simulink model "momentumBasedFlying"  (R2021b)
settings: Solver=FixedStepAuto  StartTime=0.0  StopTime=Config.simulationTime  FixedStep=Config.tStep  RelTol=1e-3
InitFcn:
  | cd(fileparts(which(bdroot)));
  | initMomentumBasedFlying;
StopFcn:
  | cd(fileparts(which(bdroot)));
  | stopMomentumBasedFlying;
undefined symbols (not defined in the file or in its folder): biasVectorConstraint_feet, Config, confVisualizer, ConstraintMatrix_feet, DiscIntNeverNeededParam, jets_config
libraries: WBToolboxLibrary x75
(part 2 of 4)

== system momentumBasedFlying/FLYING CONTROLLER (CORE) V2.5/Flight Controller RAL-HUMANOIDS V3.1- Aerodynamic Effects Compensation/Momentum Control for Flying ==
  stateMachineQuantitites : Inport
  gainsAndReferences : Inport  Port=2
  systemState : Inport  Port=3
  kinematics : Inport  Port=4
  dynamics : Inport  Port=5
  aerodynamic_force : Inport  Port=6
  Bus Selector : BusSelector  OutputSignals=jetsIntensities
  Feedback linearization : Subsystem
  Momentum Control : Subsystem
  QP Solver and Integrate Contact Forces Derivative : Subsystem
  extendedKalmanFilter4jets : Subsystem
  jointVel_star : Outport  VectorParamsAs1DForOutWhenUnconnected=off
  contactForces_star : Outport  Port=2  VectorParamsAs1DForOutWhenUnconnected=off
  jetsIntensitiesDot_star : Outport  Port=3  VectorParamsAs1DForOutWhenUnconnected=off
  "jets_throttle " : Outport  Port=4  VectorParamsAs1DForOutWhenUnconnected=off
  wires:
  QP Solver and Integrate Contact Forces Derivative/3(jointVel_star) -> jointVel_star/1
  QP Solver and Integrate Contact Forces Derivative/1(contactForces_star) -> contactForces_star/1, Momentum Control/1(contactForces_hat)  "WARNING! estimated contact forces are assumed to be coincident with contactForces_star"
  Momentum Control/4(uppeBoundQP) -> QP Solver and Integrate Contact Forces Derivative/4(upperBoundQP)
  Momentum Control/3(lowerBoundQP) -> QP Solver and Integrate Contact Forces Derivative/3(lowerBoundQP)
  Momentum Control/2(gVectorQP) -> QP Solver and Integrate Contact Forces Derivative/2(gVectorQP)
  Momentum Control/1(HessianMatrixQP) -> QP Solver and Integrate Contact Forces Derivative/1(HessianMatrixQP)
  stateMachineQuantitites/1 -> QP Solver and Integrate Contact Forces Derivative/5(stateMachineQuantities), Momentum Control/6(stateMachineQuantitites)
  gainsAndReferences/1 -> Momentum Control/5(gainsAndReferences)
  dynamics/1 -> Momentum Control/4(dynamics)
  kinematics/1 -> Momentum Control/3(kinematics)
  systemState/1 -> Bus Selector/1, QP Solver and Integrate Contact Forces Derivative/6(systemState), Momentum Control/2(systemState)
  Feedback linearization/1(throttle) -> extendedKalmanFilter4jets/2("jetsThrottle "), "jets_throttle "/1
  Bus Selector/1 -> extendedKalmanFilter4jets/1("jetsIntensityMeasured ")  "<jetsIntensities>"
  extendedKalmanFilter4jets/1(jetsState) -> Feedback linearization/1(jetState)
  QP Solver and Integrate Contact Forces Derivative/2(jetsIntensitiesDot_star) -> jetsIntensitiesDot_star/1, Feedback linearization/2(jetDerivatives_des)
  aerodynamic_force/1 -> Momentum Control/7(aerodynamic_force)

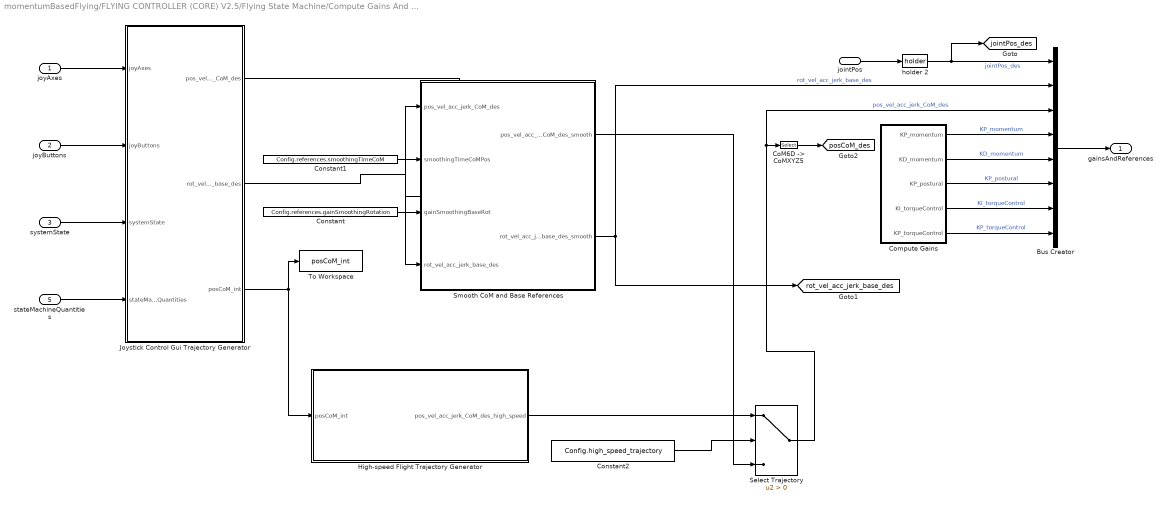
== system momentumBasedFlying/FLYING CONTROLLER (CORE) V2.5/Flying State Machine/Compute Gains And References ==
  joyAxes : Inport
  joyButtons : Inport  Port=2
  systemState : Inport  Port=3
  jointPos : Inport  Port=4
  stateMachineQuantities : Inport  Port=5
  Bus Creator : BusCreator  Inputs=8
  "CoM6D -> CoMXYZ5" : Selector  NumberOfDimensions=2  InputPortWidth=7  IndexOptions=Index vector (dialog),Index vector (dialog)  Indices=[1 2 3],[1]  OutputSizes=1,1
  Compute Gains : Subsystem
  Constant : Constant  Value=Config.references.gainSmoothingRotation
  Constant1 : Constant  Value=Config.references.smoothingTimeCoM
  Constant2 : Constant  Value=Config.high_speed_trajectory
  High-speed Flight Trajectory Generator : Subsystem
  Joystick Control Gui Trajectory Generator : Subsystem
  Select Trajectory : Switch  Criteria=u2 > Threshold
  Smooth CoM and Base References : Subsystem
  To Workspace : ToWorkspace  VariableName=posCoM_int  SaveFormat=Timeseries  SampleTime=-1
  holder 2 : WBToolboxLibrary/Utilities/holder 
      settings: SourceProductName=WholeBodyToolbox
  gainsAndReferences : Outport  VectorParamsAs1DForOutWhenUnconnected=off
  tag scope: jointPos_des=global, posCoM_des=global, rot_vel_acc_jerk_base_des=global
  wires:
  "CoM6D -> CoMXYZ5"/1 -> [posCoM_des]
  Constant1/1 -> Smooth CoM and Base References/2(smoothingTimeCoMPos)
  Smooth CoM and Base References/2(rot_vel_acc_jerk_base_des_smooth) -> [rot_vel_acc_jerk_base_des], Bus Creator/2  "rot_vel_acc_jerk_base_des"
  Compute Gains/5(KP_torqueControl) -> Bus Creator/8  "KP_torqueControl"
  Compute Gains/2(KD_momentum) -> Bus Creator/5  "KD_momentum"
  Compute Gains/1(KP_momentum) -> Bus Creator/4  "KP_momentum"
  Compute Gains/3(KP_postural) -> Bus Creator/6  "KP_postural"
  Constant/1 -> Smooth CoM and Base References/3(gainSmoothingBaseRot)
  Bus Creator/1 -> gainsAndReferences/1
  Compute Gains/4(KI_torqueControl) -> Bus Creator/7  "KI_torqueControl"
  holder 2/1 -> Bus Creator/1, [jointPos_des]  "jointPos_des"
  jointPos/1 -> holder 2/1
  joyAxes/1 -> Joystick Control Gui Trajectory Generator/1(joyAxes)
  joyButtons/1 -> Joystick Control Gui Trajectory Generator/2(joyButtons)
  systemState/1 -> Joystick Control Gui Trajectory Generator/3(systemState)
  stateMachineQuantities/1 -> Joystick Control Gui Trajectory Generator/4(stateMachineQuantities)
  Joystick Control Gui Trajectory Generator/1(pos_vel_acc_jerk_CoM_des) -> Smooth CoM and Base References/1(pos_vel_acc_jerk_CoM_des)
  Joystick Control Gui Trajectory Generator/2(rot_vel_acc_jerk_base_des) -> Smooth CoM and Base References/4(rot_vel_acc_jerk_base_des)
  High-speed Flight Trajectory Generator/1(pos_vel_acc_jerk_CoM_des_high_speed) -> Select Trajectory/1
  Smooth CoM and Base References/1(pos_vel_acc_jerk_CoM_des_smooth) -> Select Trajectory/3
  Constant2/1 -> Select Trajectory/2
  Select Trajectory/1 -> Bus Creator/3, "CoM6D -> CoMXYZ5"/1  "pos_vel_acc_jerk_CoM_des"
  Joystick Control Gui Trajectory Generator/3(posCoM_int) -> To Workspace/1, High-speed Flight Trajectory Generator/1(posCoM_int)

== system momentumBasedFlying/FLYING CONTROLLER (CORE) V2.5/Flying State Machine/Take Off//Landing State Detector ==
  systemState : Inport
  joyButtons : Inport  Port=2
  Bus Creator : BusCreator  Inputs=6
  Bus Selector : BusSelector  OutputSignals=contactForces
  Demux : Demux  Outputs=[6;6]
  MATLAB Function : MATLAB Function  TreatAsAtomicUnit=on
  Vertical Forces Control : MATLAB Function  TreatAsAtomicUnit=on
  stateMachineQuantities : Outport  VectorParamsAs1DForOutWhenUnconnected=off
  tag scope: stateMachineQuantities=global
  wires:
  Vertical Forces Control/1(decreaseMaxFootVerticalForce) -> Bus Creator/1  "decreaseMaxFootVerticalForce"
  Vertical Forces Control/2(increaseMinFootVerticalForce) -> Bus Creator/2  "increaseMinFootVerticalForce"
  Bus Creator/1 -> [stateMachineQuantities], stateMachineQuantities/1
  systemState/1 -> Bus Selector/1
  joyButtons/1 -> Vertical Forces Control/1(joyButtons)
  Demux/2 -> MATLAB Function/2(wrench_r)
  Demux/1 -> MATLAB Function/1(wrench_l)
  Bus Selector/1 -> Demux/1  "<contactForces>"
  MATLAB Function/1(feetContactIsActive) -> Bus Creator/4  "feetContactIsActive"
  MATLAB Function/2(robotIsLanded) -> Bus Creator/5  "robotIsLanded"
  MATLAB Function/3(oneFootIsInContact) -> Bus Creator/6  "oneFootIsInContact"
  Vertical Forces Control/3(activateEqConstrTorqueControl) -> Bus Creator/3  "activateEqConstrTorqueControl"

== system momentumBasedFlying/FLYING CONTROLLER (CORE) V2.5/Get System State/Change Contact Forces Representation ==
  jointPos : Inport
  w_H_b : Inport  Port=2
  contactForces_WBD : Inport  Port=3
  Change Contact Forces Representation : MATLAB Function  TreatAsAtomicUnit=on
  "CoM6D -> CoMXYZ1" : Selector  NumberOfDimensions=2  InputPortWidth=7  IndexOptions=Index vector (dialog),Index vector (dialog)  Indices=[1 2 3],[1 2 3]  OutputSizes=1,1
  "CoM6D -> CoMXYZ3" : Selector  NumberOfDimensions=2  InputPortWidth=7  IndexOptions=Index vector (dialog),Index vector (dialog)  Indices=[1 2 3],[1 2 3]  OutputSizes=1,1
  LFoot Pose : WBToolboxLibrary/Model/Kinematics/ForwardKinematics  frameName=Frames.LFOOT_FRAME
      settings: SourceProductName=WholeBodyToolbox
  Mux : Mux  Inputs=2
  RFoot Pose : WBToolboxLibrary/Model/Kinematics/ForwardKinematics  frameName=Frames.RFOOT_FRAME
      settings: SourceProductName=WholeBodyToolbox
  contactForces : Outport  VectorParamsAs1DForOutWhenUnconnected=off
  tag scope: wrench_LFoot=global, wrench_RFoot=global
  wires:
  contactForces_WBD/1 -> Change Contact Forces Representation/1(contactForces_WBD)
  RFoot Pose/1 -> "CoM6D -> CoMXYZ3"/1
  "CoM6D -> CoMXYZ3"/1 -> Change Contact Forces Representation/3(w_R_r_sole)
  LFoot Pose/1 -> "CoM6D -> CoMXYZ1"/1
  "CoM6D -> CoMXYZ1"/1 -> Change Contact Forces Representation/2(w_R_l_sole)
  w_H_b/1 -> LFoot Pose/1, RFoot Pose/1
  jointPos/1 -> LFoot Pose/2, RFoot Pose/2
  Change Contact Forces Representation/1(mixed_f_l_sole) -> [wrench_LFoot], Mux/1
  Change Contact Forces Representation/2(mixed_f_r_sole) -> [wrench_RFoot], Mux/2
  Mux/1 -> contactForces/1

== system momentumBasedFlying/Visualizer/Task and Base Frame Kinematics/Combine Rotations ==
  roll : Inport
  pitch : Inport  Port=2
  yaw : Inport  Port=3
  roll_des : Inport  Port=4
  pitch_des : Inport  Port=5
  yaw_des : Inport  Port=6
  Mux : Mux  Inputs=2
  Mux1 : Mux  Inputs=2
  Mux2 : Mux  Inputs=2
  Task rotation combined : Scope  NumInputPorts=3
  wires:
  yaw_des/1 -> Mux2/2
  pitch_des/1 -> Mux1/2
  pitch/1 -> Mux1/1
  roll/1 -> Mux/1
  yaw/1 -> Mux2/1
  roll_des/1 -> Mux/2
  Mux2/1 -> Task rotation combined/3
  Mux1/1 -> Task rotation combined/2
  Mux/1 -> Task rotation combined/1

== system momentumBasedFlying/iRonCub/Forward Dynamics/aerodynamic visualizer ==
  aerodynamic_forces_total : Inport
  relative_velocity : Inport  Port=2
  alpha : Inport  Port=3
  beta : Inport  Port=4
  drag_force : Inport  Port=5
  normal_force : Inport  Port=6
  Scope : Scope
  Scope1 : Scope
  Scope2 : Scope
  To Workspace : ToWorkspace  VariableName=Fa_drag  SaveFormat=Timeseries  SampleTime=-1
  To Workspace1 : ToWorkspace  VariableName=Fa_normal  SaveFormat=Timeseries  SampleTime=-1
  To Workspace2 : ToWorkspace  VariableName=Fa  SaveFormat=Timeseries  SampleTime=-1
  To Workspace3 : ToWorkspace  VariableName=Va  SaveFormat=Timeseries  SampleTime=-1
  To Workspace4 : ToWorkspace  VariableName=alpha  SaveFormat=Timeseries  SampleTime=-1
  To Workspace5 : ToWorkspace  VariableName=beta  SaveFormat=Timeseries  SampleTime=-1
  r : Scope
  wires:
  beta/1 -> Scope2/1, To Workspace5/1
  relative_velocity/1 -> r/1, To Workspace3/1
  aerodynamic_forces_total/1 -> Scope1/1, To Workspace2/1
  alpha/1 -> Scope/1, To Workspace4/1
  drag_force/1 -> To Workspace/1
  normal_force/1 -> To Workspace1/1

== system momentumBasedFlying/FLYING CONTROLLER (CORE) V2.5/Dynamics and Kinematics/Dynamic Quantities/Compute Centroidal Inertia ==
  M : Inport
  w_H_b : Inport  Port=2
  posCoM : Inport  Port=3
  Compute Centroidal Inertia : MATLAB Function  TreatAsAtomicUnit=on
  Selector : Selector  NumberOfDimensions=2  InputPortWidth=3  IndexOptions=Index vector (dialog),Index vector (dialog)  Indices=[1 2 3],4  OutputSizes=1,1
  w_I_c : Outport  VectorParamsAs1DForOutWhenUnconnected=off
  wires:
  M/1 -> Compute Centroidal Inertia/1(M)
  w_H_b/1 -> Selector/1
  Selector/1 -> Compute Centroidal Inertia/3(posBase)
  posCoM/1 -> Compute Centroidal Inertia/2(posCoM)
  Compute Centroidal Inertia/1(w_I_c) -> w_I_c/1

== system momentumBasedFlying/FLYING CONTROLLER (CORE) V2.5/Dynamics and Kinematics/Dynamic Quantities/Momentum and CentroidalMomentum Matrix ==
  w_H_b : Inport
  jointPos : Inport  Port=2
  w_baseTwist : Inport  Port=3
  jointVel : Inport  Port=4
  CentroidalMomentum : WBToolboxLibrary/Model/Dynamics/CentroidalMomentum
      settings: SourceProductName=WholeBodyToolbox
  CentroidalMomentum Matrix iCub 23/25 DoFs : Subsystem
  L : Outport  VectorParamsAs1DForOutWhenUnconnected=off
  CMM : Outport  Port=2  VectorParamsAs1DForOutWhenUnconnected=off
  wires:
  w_baseTwist/1 -> CentroidalMomentum/3
  CentroidalMomentum/1 -> L/1
  w_H_b/1 -> CentroidalMomentum Matrix iCub 23/25 DoFs/1(w_H_b), CentroidalMomentum/1
  jointPos/1 -> CentroidalMomentum Matrix iCub 23/25 DoFs/2(jointPos), CentroidalMomentum/2
  jointVel/1 -> CentroidalMomentum/4
  CentroidalMomentum Matrix iCub 23/25 DoFs/1(CMM) -> CMM/1

== system momentumBasedFlying/FLYING CONTROLLER (CORE) V2.5/Dynamics and Kinematics/Kinematic Quantities/Compute Thrusts Axes and Arms ==
  posCoM : Inport
  w_H_b : Inport  Port=2
  jointPos : Inport  Port=3
  Pose Jet 1 : WBToolboxLibrary/Model/Kinematics/ForwardKinematics  frameName=Frames.JET1_FRAME
      settings: SourceProductName=WholeBodyToolbox
  Pose Jet 2 : WBToolboxLibrary/Model/Kinematics/ForwardKinematics  frameName=Frames.JET2_FRAME
      settings: SourceProductName=WholeBodyToolbox
  Pose Jet 3 : WBToolboxLibrary/Model/Kinematics/ForwardKinematics  frameName=Frames.JET3_FRAME
      settings: SourceProductName=WholeBodyToolbox
  Pose Jet 4 : WBToolboxLibrary/Model/Kinematics/ForwardKinematics  frameName=Frames.JET4_FRAME
      settings: SourceProductName=WholeBodyToolbox
  Thrust Axes and Arms : MATLAB Function  TreatAsAtomicUnit=on
  matrixOfJetsAxes : Outport  VectorParamsAs1DForOutWhenUnconnected=off
  matrixOfJetsArms : Outport  Port=2  VectorParamsAs1DForOutWhenUnconnected=off
  wires:
  Pose Jet 2/1 -> Thrust Axes and Arms/2(w_H_J2)
  jointPos/1 -> Pose Jet 1/2, Pose Jet 2/2, Pose Jet 3/2, Pose Jet 4/2
  Pose Jet 1/1 -> Thrust Axes and Arms/1(w_H_J1)
  Pose Jet 3/1 -> Thrust Axes and Arms/3(w_H_J3)
  Pose Jet 4/1 -> Thrust Axes and Arms/4(w_H_J4)
  Thrust Axes and Arms/1(matrixOfJetsAxes) -> matrixOfJetsAxes/1
  Thrust Axes and Arms/2(matrixOfJetsArms) -> matrixOfJetsArms/1
  w_H_b/1 -> Pose Jet 4/1, Pose Jet 3/1, Pose Jet 2/1, Pose Jet 1/1
  posCoM/1 -> Thrust Axes and Arms/5(posCoM)

== system momentumBasedFlying/FLYING CONTROLLER (CORE) V2.5/Flight Controller RAL-HUMANOIDS V3.1- Aerodynamic Effects Compensation/Joint Torque Control for Flying/Integrate Joints Velocity error ==
  jointVel_err : Inport
  Constant : Constant  Value=zeros(Config.N_DOF,1)
  Discrete-Time Integrator1 : DiscreteIntegrator  InitialConditionSource=external  InitialCondition=zeros(Config.N_DOF,1)  SampleTime=Config.tStep  ICPrevOutput=DiscIntNeverNeededParam  ICPrevScaledInput=DiscIntNeverNeededParam
  jointPos_err : Outport  VectorParamsAs1DForOutWhenUnconnected=off
  tag scope: jointPos_err_integral=global
  wires:
  Constant/1 -> Discrete-Time Integrator1/2
  jointVel_err/1 -> Discrete-Time Integrator1/1
  Discrete-Time Integrator1/1 -> [jointPos_err_integral], jointPos_err/1

== system momentumBasedFlying/FLYING CONTROLLER (CORE) V2.5/Flight Controller RAL-HUMANOIDS V3.1- Aerodynamic Effects Compensation/Joint Torque Control for Flying/QP torqueControl ==
  HessianMatrixQP : Inport
  gVectorQP : Inport  Port=2
  ConstraintMatrix_inequality : Inport  Port=3
  biasVectorConstraint_inequality : Inport  Port=4
  feetContactIsActive : Inport  Port=5
  Constant2 : Constant  Value=Config.sat.jointTorquesSaturation
  NOT : Logic  Operator=NOT  IconShape=distinctive  AllPortsSameDT=off  OutDataTypeStr=boolean
  Process QP Inputs Torque Control : MATLAB Function  TreatAsAtomicUnit=on
  QP torqueControl - balancing : Subsystem  TreatAsAtomicUnit=on
  QP torqueControl - flight : Subsystem  TreatAsAtomicUnit=on
  Select QP torqueControl Output : Subsystem
  jointTorques_star : Outport  VectorParamsAs1DForOutWhenUnconnected=off
  exitFlagQP_torqueControl : Outport  Port=2  VectorParamsAs1DForOutWhenUnconnected=off
  wires:
  Select QP torqueControl Output/1(jointTorques_star) -> jointTorques_star/1
  Select QP torqueControl Output/2(exitFlagQP_torqueControl) -> exitFlagQP_torqueControl/1
  QP torqueControl - flight/1(QPStatus_flight) -> Select QP torqueControl Output/4(QPStatus_flight)
  QP torqueControl - flight/2(QPOutput_flight) -> Select QP torqueControl Output/5(QPOutput_flight)
  QP torqueControl - balancing/2(QPOutput_balancing) -> Select QP torqueControl Output/2(QPOutput_balancing)
  QP torqueControl - balancing/1(QPStatus_balancing) -> Select QP torqueControl Output/1(QPStatus_balancing)
  Process QP Inputs Torque Control/1(H_balancing) -> QP torqueControl - balancing/1(H)
  Process QP Inputs Torque Control/2(g_balancing) -> QP torqueControl - balancing/2(g)
  Process QP Inputs Torque Control/3(ub_balancing) -> QP torqueControl - balancing/3(ub)
  Process QP Inputs Torque Control/4(lb_balancing) -> QP torqueControl - balancing/4(lb)
  Process QP Inputs Torque Control/5(Aeq_balancing) -> QP torqueControl - balancing/5(AEq)
  Process QP Inputs Torque Control/6(lbEq_balancing) -> QP torqueControl - balancing/6(lbEq)
  Process QP Inputs Torque Control/7(ubEq_balancing) -> QP torqueControl - balancing/7(ubEq)
  Process QP Inputs Torque Control/11(lb_flight) -> QP torqueControl - flight/4(lb)
  Process QP Inputs Torque Control/10(ub_flight) -> QP torqueControl - flight/3(ub)
  Process QP Inputs Torque Control/9(g_flight) -> QP torqueControl - flight/2(g)
  Process QP Inputs Torque Control/8(H_flight) -> QP torqueControl - flight/1(H)
  Constant2/1 -> Process QP Inputs Torque Control/5(jointTorquesSaturation)
  gVectorQP/1 -> Process QP Inputs Torque Control/2(gVectorQP)
  HessianMatrixQP/1 -> Process QP Inputs Torque Control/1(HessianMatrixQP)
  ConstraintMatrix_inequality/1 -> Process QP Inputs Torque Control/3(InequalityConstrMatrix)
  biasVectorConstraint_inequality/1 -> Process QP Inputs Torque Control/4(biasVectorInequalityConstr)
  NOT/1 -> QP torqueControl - flight/Enable
  feetContactIsActive/1 -> NOT/1, QP torqueControl - balancing/Enable, Select QP torqueControl Output/3(feetContactIsActive)

== system momentumBasedFlying/FLYING CONTROLLER (CORE) V2.5/Flight Controller RAL-HUMANOIDS V3.1- Aerodynamic Effects Compensation/Joint Torque Control for Flying/Torque Derivative Saturation ==
  jointTorques_star : Inport
  Constant1 : Constant  Value=Config.tStep
  Constant2 : Constant  Value=Config.sat.jointTorquesDotMax
  Saturate Torque Derivative : MATLAB Function  TreatAsAtomicUnit=on
  "holder " : WBToolboxLibrary/Utilities/holder 
      settings: SourceProductName=WholeBodyToolbox
  jointTorques_star_sat : Outport  VectorParamsAs1DForOutWhenUnconnected=off
  wires:
  Constant2/1 -> Saturate Torque Derivative/4(uDotMax)
  Constant1/1 -> Saturate Torque Derivative/3(tStep)
  "holder "/1 -> Saturate Torque Derivative/2(u_0)
  Saturate Torque Derivative/1(uSat) -> jointTorques_star_sat/1
  jointTorques_star/1 -> Saturate Torque Derivative/1(u), "holder "/1

== system momentumBasedFlying/FLYING CONTROLLER (CORE) V2.5/Flight Controller RAL-HUMANOIDS V3.1- Aerodynamic Effects Compensation/Momentum Control for Flying/Feedback linearization ==
  jetState : Inport
  jetDerivatives_des : Inport  Port=2
  Bus Selector : BusSelector  OutputSignals=jetIntensitiesFiltered,jetDerivativesEst
  Discrete-Time Integrator : DiscreteIntegrator  SampleTime=Config.tStep  ICPrevOutput=DiscIntNeverNeededParam  ICPrevScaledInput=DiscIntNeverNeededParam
  Error : Scope
  MATLAB Function : MATLAB Function  TreatAsAtomicUnit=on
  jetDerivatives : Scope  NumInputPorts=3
  throttle : Outport  VectorParamsAs1DForOutWhenUnconnected=off
  wires:
  Bus Selector/1 -> MATLAB Function/1(jets)  "<jetIntensitiesFiltered>"
  MATLAB Function/1(throttle) -> jetDerivatives/1, throttle/1  "throttle"
  jetState/1 -> Bus Selector/1
  MATLAB Function/2(error) -> Error/1, Discrete-Time Integrator/1  "error"
  Bus Selector/2 -> jetDerivatives/3, MATLAB Function/2(jets_dot)  "<jetDerivativesEst>"
  Discrete-Time Integrator/1 -> MATLAB Function/4(integral_err)
  jetDerivatives_des/1 -> MATLAB Function/3(jets_dot_des), jetDerivatives/2

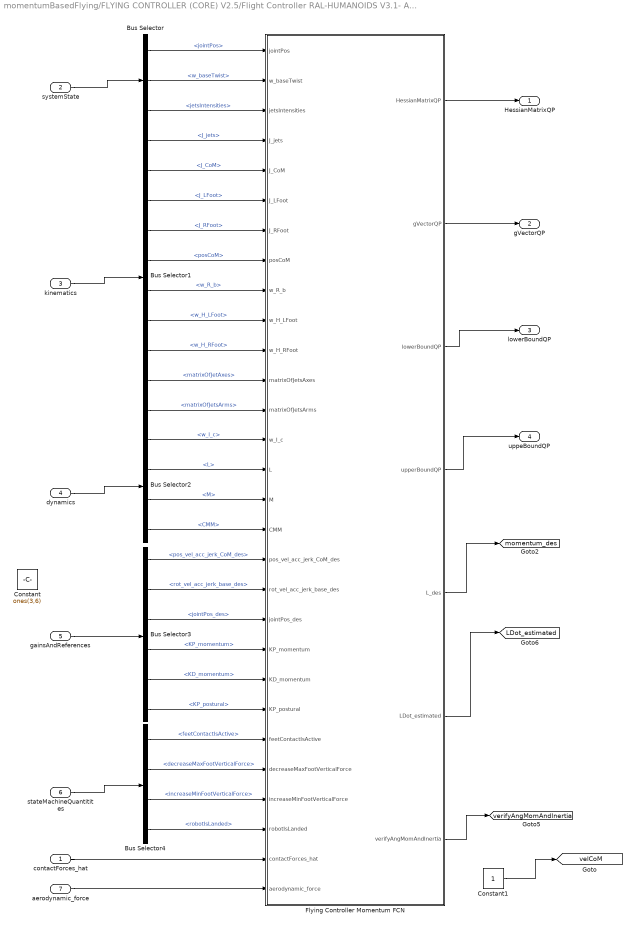
== system momentumBasedFlying/FLYING CONTROLLER (CORE) V2.5/Flight Controller RAL-HUMANOIDS V3.1- Aerodynamic Effects Compensation/Momentum Control for Flying/Momentum Control ==
  contactForces_hat : Inport
  systemState : Inport  Port=2
  kinematics : Inport  Port=3
  dynamics : Inport  Port=4
  gainsAndReferences : Inport  Port=5
  stateMachineQuantitites : Inport  Port=6
  aerodynamic_force : Inport  Port=7
  Bus Selector : BusSelector  OutputSignals=jointPos,w_baseTwist,jetsIntensities
  Bus Selector1 : BusSelector  OutputSignals=J_jets,J_CoM,J_LFoot,J_RFoot,posCoM,w_R_b,w_H_LFoot,w_H_RFoot,matrixOfJetAxes,matrixOfJetsArms
  Bus Selector2 : BusSelector  OutputSignals=w_I_c,L,M,CMM
  Bus Selector3 : BusSelector  OutputSignals=pos_vel_acc_jerk_CoM_des,rot_vel_acc_jerk_base_des,jointPos_des,KP_momentum,KD_momentum,KP_postural
  Bus Selector4 : BusSelector  OutputSignals=feetContactIsActive,decreaseMaxFootVerticalForce,increaseMinFootVerticalForce,robotIsLanded
  Constant : Constant  Value=ones(3,6)
  Constant1 : Constant
  "Flying Controller Momentum FCN " : MATLAB Function  TreatAsAtomicUnit=on
  HessianMatrixQP : Outport  VectorParamsAs1DForOutWhenUnconnected=off
  gVectorQP : Outport  Port=2  VectorParamsAs1DForOutWhenUnconnected=off
  lowerBoundQP : Outport  Port=3  VectorParamsAs1DForOutWhenUnconnected=off
  uppeBoundQP : Outport  Port=4  VectorParamsAs1DForOutWhenUnconnected=off
  tag scope: LDot_estimated=global, momentum_des=global, velCoM=global, verifyAngMomAndInertia=global
  wires:
  Constant1/1 -> [velCoM]
  contactForces_hat/1 -> "Flying Controller Momentum FCN "/28(contactForces_hat)
  Bus Selector4/4 -> "Flying Controller Momentum FCN "/27(robotIsLanded)  "<robotIsLanded>"
  Bus Selector4/3 -> "Flying Controller Momentum FCN "/26(increaseMinFootVerticalForce)  "<increaseMinFootVerticalForce>"
  Bus Selector4/2 -> "Flying Controller Momentum FCN "/25(decreaseMaxFootVerticalForce)  "<decreaseMaxFootVerticalForce>"
  Bus Selector2/1 -> "Flying Controller Momentum FCN "/14(w_I_c)  "<w_I_c>"
  Bus Selector1/10 -> "Flying Controller Momentum FCN "/13(matrixOfJetsArms)  "<matrixOfJetsArms>"
  Bus Selector1/9 -> "Flying Controller Momentum FCN "/12(matrixOfJetsAxes)  "<matrixOfJetAxes>"
  Bus Selector3/1 -> "Flying Controller Momentum FCN "/18(pos_vel_acc_jerk_CoM_des)  "<pos_vel_acc_jerk_CoM_des>"
  Bus Selector1/6 -> "Flying Controller Momentum FCN "/9(w_R_b)  "<w_R_b>"
  Bus Selector1/5 -> "Flying Controller Momentum FCN "/8(posCoM)  "<posCoM>"
  "Flying Controller Momentum FCN "/5(L_des) -> [momentum_des]
  Bus Selector3/6 -> "Flying Controller Momentum FCN "/23(KP_postural)  "<KP_postural>"
  Bus Selector2/2 -> "Flying Controller Momentum FCN "/15(L)  "<L>"
  Bus Selector1/7 -> "Flying Controller Momentum FCN "/10(w_H_LFoot)  "<w_H_LFoot>"
  Bus Selector3/5 -> "Flying Controller Momentum FCN "/22(KD_momentum)  "<KD_momentum>"
  "Flying Controller Momentum FCN "/6(LDot_estimated) -> [LDot_estimated]
  Bus Selector2/3 -> "Flying Controller Momentum FCN "/16(M)  "<M>"
  Bus Selector2/4 -> "Flying Controller Momentum FCN "/17(CMM)  "<CMM>"
  Bus Selector1/8 -> "Flying Controller Momentum FCN "/11(w_H_RFoot)  "<w_H_RFoot>"
  Bus Selector1/4 -> "Flying Controller Momentum FCN "/7(J_RFoot)  "<J_RFoot>"
  Bus Selector/3 -> "Flying Controller Momentum FCN "/3(jetsIntensities)  "<jetsIntensities>"
  gainsAndReferences/1 -> Bus Selector3/1
  Bus Selector1/2 -> "Flying Controller Momentum FCN "/5(J_CoM)  "<J_CoM>"
  dynamics/1 -> Bus Selector2/1
  Bus Selector3/4 -> "Flying Controller Momentum FCN "/21(KP_momentum)  "<KP_momentum>"
  "Flying Controller Momentum FCN "/3(lowerBoundQP) -> lowerBoundQP/1
  stateMachineQuantitites/1 -> Bus Selector4/1
  "Flying Controller Momentum FCN "/7(verifyAngMomAndInertia) -> [verifyAngMomAndInertia]
  Bus Selector4/1 -> "Flying Controller Momentum FCN "/24(feetContactIsActive)  "<feetContactIsActive>"
  "Flying Controller Momentum FCN "/2(gVectorQP) -> gVectorQP/1
  "Flying Controller Momentum FCN "/4(upperBoundQP) -> uppeBoundQP/1
  "Flying Controller Momentum FCN "/1(HessianMatrixQP) -> HessianMatrixQP/1
  Bus Selector/2 -> "Flying Controller Momentum FCN "/2(w_baseTwist)  "<w_baseTwist>"
  Bus Selector1/1 -> "Flying Controller Momentum FCN "/4(J_jets)  "<J_jets>"
  Bus Selector/1 -> "Flying Controller Momentum FCN "/1(jointPos)  "<jointPos>"
  kinematics/1 -> Bus Selector1/1
  Bus Selector1/3 -> "Flying Controller Momentum FCN "/6(J_LFoot)  "<J_LFoot>"
  Bus Selector3/3 -> "Flying Controller Momentum FCN "/20(jointPos_des)  "<jointPos_des>"
  systemState/1 -> Bus Selector/1
  Bus Selector3/2 -> "Flying Controller Momentum FCN "/19(rot_vel_acc_jerk_base_des)  "<rot_vel_acc_jerk_base_des>"
  aerodynamic_force/1 -> "Flying Controller Momentum FCN "/29(aerodynamic_force)

== system momentumBasedFlying/FLYING CONTROLLER (CORE) V2.5/Flight Controller RAL-HUMANOIDS V3.1- Aerodynamic Effects Compensation/Momentum Control for Flying/QP Solver and Integrate Contact Forces Derivative ==
  HessianMatrixQP : Inport
  gVectorQP : Inport  Port=2
  lowerBoundQP : Inport  Port=3
  upperBoundQP : Inport  Port=4
  stateMachineQuantities : Inport  Port=5
  systemState : Inport  Port=6
  Bus Selector1 : BusSelector  OutputSignals=feetContactIsActive
  Bus Selector2 : BusSelector  OutputSignals=contactForces
  Integrate the Contact Forces Derivative : Subsystem
  QP momentumControl : Subsystem
  contactForces_star : Outport  VectorParamsAs1DForOutWhenUnconnected=off
  jetsIntensitiesDot_star : Outport  Port=2  VectorParamsAs1DForOutWhenUnconnected=off
  jointVel_star : Outport  Port=3  VectorParamsAs1DForOutWhenUnconnected=off
  tag scope: contactForces_star=global, exitFlagQP_momentumControl=global, jetsIntensitiesDot_star=global, jointVel_star=global
  wires:
  systemState/1 -> Bus Selector2/1
  Bus Selector2/1 -> Integrate the Contact Forces Derivative/2(contactForces)  "<contactForces>"
  Bus Selector1/1 -> Integrate the Contact Forces Derivative/3(feetContactIsActive), QP momentumControl/5(feetContactIsActive)  "<feetContactIsActive>"
  QP momentumControl/3(jointVel_star) -> jointVel_star/1, [jointVel_star]
  QP momentumControl/1(jetsIntensitiesDot_star) -> jetsIntensitiesDot_star/1, [jetsIntensitiesDot_star]
  HessianMatrixQP/1 -> QP momentumControl/1(HessianMatrixQP)
  stateMachineQuantities/1 -> Bus Selector1/1
  gVectorQP/1 -> QP momentumControl/2(gVectorQP)
  QP momentumControl/4(exitFlagQP_momentumControl) -> [exitFlagQP_momentumControl]
  upperBoundQP/1 -> QP momentumControl/4(upperBoundQP)
  lowerBoundQP/1 -> QP momentumControl/3(lowerBoundQP)
  Integrate the Contact Forces Derivative/1(contactForces_star) -> contactForces_star/1, [contactForces_star]
  QP momentumControl/2(contactForcesDot_star) -> Integrate the Contact Forces Derivative/1(contactForcesDot_star)

== system momentumBasedFlying/FLYING CONTROLLER (CORE) V2.5/Flight Controller RAL-HUMANOIDS V3.1- Aerodynamic Effects Compensation/Momentum Control for Flying/extendedKalmanFilter4jets ==
  "jetsIntensityMeasured " : Inport
  "jetsThrottle " : Inport  Port=2
  Bus Creator : BusCreator  Inputs=2
  Demux : Demux
  Demux1 : Demux
  EKF_jet1 : Subsystem
  EKF_jet2 : Subsystem
  EKF_jet3 : Subsystem
  EKF_jet4 : Subsystem
  Mux : Mux
  Mux1 : Mux
  jetsState : Outport
  wires:
  Demux/1 -> EKF_jet1/1(input)
  Demux/2 -> EKF_jet2/1(input)
  Demux/3 -> EKF_jet3/1(input)
  Demux/4 -> EKF_jet4/1(input)
  Demux1/1 -> EKF_jet1/2(jetIntensityMeasurement)
  Demux1/2 -> EKF_jet2/2(jetIntensityMeasurement)
  Demux1/3 -> EKF_jet3/2(jetIntensityMeasurement)
  Demux1/4 -> EKF_jet4/2(jetIntensityMeasurement)
  EKF_jet2/1(jetIntensityFiltered) -> Mux/2
  EKF_jet1/1(jetIntensityFiltered) -> Mux/1
  EKF_jet3/1(jetIntensityFiltered) -> Mux/3
  EKF_jet4/1(jetIntensityFiltered) -> Mux/4
  EKF_jet1/2(jetDerivativeEstimated) -> Mux1/1
  EKF_jet2/2(jetDerivativeEstimated) -> Mux1/2
  EKF_jet3/2(jetDerivativeEstimated) -> Mux1/3
  EKF_jet4/2(jetDerivativeEstimated) -> Mux1/4
  "jetsThrottle "/1 -> Demux/1
  "jetsIntensityMeasured "/1 -> Demux1/1
  Mux/1 -> Bus Creator/1  "jetIntensitiesFiltered"
  Mux1/1 -> Bus Creator/2  "jetDerivativesEst"
  Bus Creator/1 -> jetsState/1

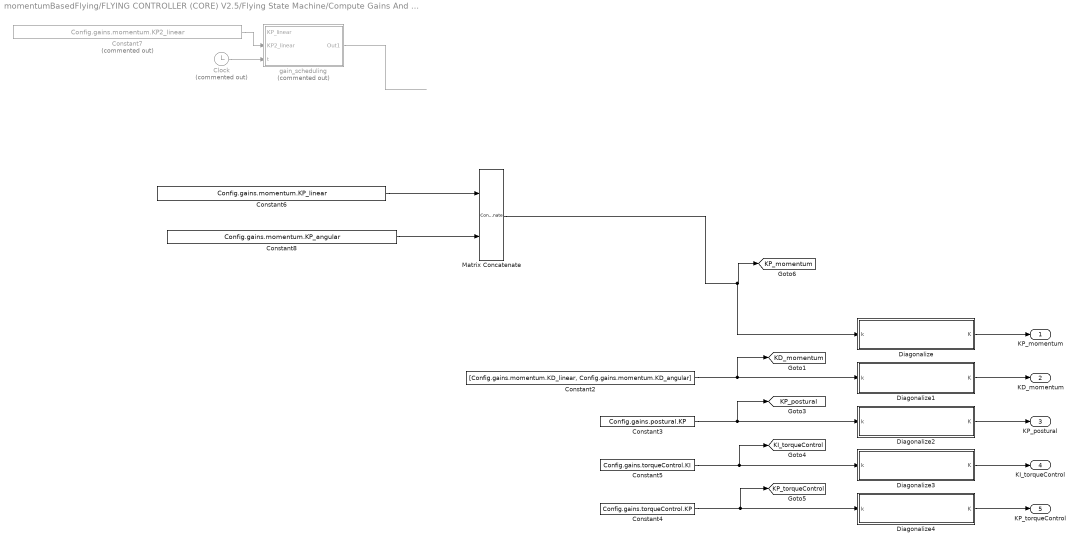
== system momentumBasedFlying/FLYING CONTROLLER (CORE) V2.5/Flying State Machine/Compute Gains And References/Compute Gains ==
  Clock : Clock  Commented=on
  Constant2 : Constant  Value=[Config.gains.momentum.KD_linear, Config.gains.momentum.KD_angular]
  Constant3 : Constant  Value=Config.gains.postural.KP
  Constant4 : Constant  Value=Config.gains.torqueControl.KP
  Constant5 : Constant  Value=Config.gains.torqueControl.KI
  Constant6 : Constant  Value=Config.gains.momentum.KP_linear
  Constant7 : Constant  Commented=on  Value=Config.gains.momentum.KP2_linear
  Constant8 : Constant  Value=Config.gains.momentum.KP_angular
  Diagonalize : MATLAB Function  TreatAsAtomicUnit=on
  Diagonalize1 : MATLAB Function  TreatAsAtomicUnit=on
  Diagonalize2 : MATLAB Function  TreatAsAtomicUnit=on
  Diagonalize3 : MATLAB Function  TreatAsAtomicUnit=on
  Diagonalize4 : MATLAB Function  TreatAsAtomicUnit=on
  Matrix Concatenate : Concatenate  ConcatenateDimension=2
  gain_scheduling : Subsystem  Commented=on
  KP_momentum : Outport  VectorParamsAs1DForOutWhenUnconnected=off
  KD_momentum : Outport  Port=2  VectorParamsAs1DForOutWhenUnconnected=off
  KP_postural : Outport  Port=3  VectorParamsAs1DForOutWhenUnconnected=off
  KI_torqueControl : Outport  Port=4  VectorParamsAs1DForOutWhenUnconnected=off
  KP_torqueControl : Outport  Port=5  VectorParamsAs1DForOutWhenUnconnected=off
  tag scope: KD_momentum=global, KI_torqueControl=global, KP_momentum=global, KP_postural=global, KP_torqueControl=global
  wires:
  Diagonalize/1(K) -> KP_momentum/1
  Diagonalize1/1(K) -> KD_momentum/1
  Diagonalize2/1(K) -> KP_postural/1
  Diagonalize3/1(K) -> KI_torqueControl/1
  Diagonalize4/1(K) -> KP_torqueControl/1
  Constant2/1 -> [KD_momentum], Diagonalize1/1(k)
  Constant3/1 -> [KP_postural], Diagonalize2/1(k)
  Constant5/1 -> [KI_torqueControl], Diagonalize3/1(k)
  Constant4/1 -> [KP_torqueControl], Diagonalize4/1(k)
  Constant8/1 -> Matrix Concatenate/2
  Matrix Concatenate/1 -> Diagonalize/1(k), [KP_momentum]
  gain_scheduling/1(Out1) -> ?
  Constant7/1 -> gain_scheduling/2(KP2_linear)
  Clock/1 -> gain_scheduling/3(t)
  Constant6/1 -> Matrix Concatenate/1

== system momentumBasedFlying/FLYING CONTROLLER (CORE) V2.5/Flying State Machine/Compute Gains And References/High-speed Flight Trajectory Generator ==
  posCoM_int : Inport
  Clock1 : Clock
  MATLAB Function : MATLAB Function  TreatAsAtomicUnit=on
  pos_vel_acc_jerk_CoM_des_high_speed : Outport
  wires:
  [posCoM] -> MATLAB Function/3(posCoM)
  posCoM_int/1 -> MATLAB Function/2(posCoM_int)
  MATLAB Function/1(pos_vel_acc_jerk_CoM_des) -> pos_vel_acc_jerk_CoM_des_high_speed/1  "pos_vel_acc_jerk_CoM_des"
  Clock1/1 -> MATLAB Function/1(t)

== system momentumBasedFlying/FLYING CONTROLLER (CORE) V2.5/Flying State Machine/Compute Gains And References/Joystick Control Gui Trajectory Generator ==
  joyAxes : Inport
  joyButtons : Inport  Port=2
  systemState : Inport  Port=3
  stateMachineQuantities : Inport  Port=4
  Bus Selector : BusSelector  OutputSignals=w_H_b,jointPos
  Bus Selector1 : BusSelector  OutputSignals=feetContactIsActive,oneFootIsInContact
  Clock : Clock
  Compute CoM and Base Rotation References : MATLAB Function  TreatAsAtomicUnit=on
  Detect Robot Movement Request From Joystick : MATLAB Function  TreatAsAtomicUnit=on
  ForwardKinematics : WBToolboxLibrary/Model/Kinematics/ForwardKinematics  frameName=Frames.COM_FRAME
      settings: SourceProductName=WholeBodyToolbox
  Selector : Selector  NumberOfDimensions=2  InputPortWidth=3  IndexOptions=Index vector (dialog),Index vector (dialog)  Indices=[1 2 3],[1 2 3]  OutputSizes=1,1
  Selector1 : Selector  NumberOfDimensions=2  InputPortWidth=3  IndexOptions=Index vector (dialog),Index vector (dialog)  Indices=[1 2 3],[4]  OutputSizes=1,1
  "holder " : WBToolboxLibrary/Utilities/holder 
      settings: SourceProductName=WholeBodyToolbox
  holder 1 : WBToolboxLibrary/Utilities/holder 
      settings: SourceProductName=WholeBodyToolbox
  pos_vel_acc_jerk_CoM_des : Outport  VectorParamsAs1DForOutWhenUnconnected=off
  rot_vel_acc_jerk_base_des : Outport  Port=2  VectorParamsAs1DForOutWhenUnconnected=off
  posCoM_int : Outport  Port=3
  wires:
  Bus Selector1/2 -> Compute CoM and Base Rotation References/12(oneFootIsInContact)  "<oneFootIsInContact>"
  Detect Robot Movement Request From Joystick/8(goLandingPos) -> Compute CoM and Base Rotation References/10(goLandingPos)
  Selector1/1 -> posCoM_int/1, Compute CoM and Base Rotation References/1(posCoM_init)
  Compute CoM and Base Rotation References/2(rot_vel_acc_jerk_base_des) -> rot_vel_acc_jerk_base_des/1
  joyButtons/1 -> Detect Robot Movement Request From Joystick/2(joyButtons)
  joyAxes/1 -> Detect Robot Movement Request From Joystick/1(joyAxes)
  systemState/1 -> Bus Selector/1
  Clock/1 -> Compute CoM and Base Rotation References/13(t)
  Detect Robot Movement Request From Joystick/6(rotateYaw) -> Compute CoM and Base Rotation References/8(rotateYaw)
  Compute CoM and Base Rotation References/1(pos_vel_acc_jerk_CoM_des) -> pos_vel_acc_jerk_CoM_des/1
  Detect Robot Movement Request From Joystick/4(rotateRoll) -> Compute CoM and Base Rotation References/6(rotateRoll)
  ForwardKinematics/1 -> "holder "/1
  holder 1/1 -> Compute CoM and Base Rotation References/2(w_R_b_init)
  Bus Selector/1 -> Selector/1, ForwardKinematics/1  "<w_H_b>"
  Selector/1 -> holder 1/1
  Bus Selector1/1 -> Compute CoM and Base Rotation References/11(feetContactIsActive)  "<feetContactIsActive>"
  Detect Robot Movement Request From Joystick/5(rotatePitch) -> Compute CoM and Base Rotation References/7(rotatePitch)
  stateMachineQuantities/1 -> Bus Selector1/1
  Detect Robot Movement Request From Joystick/2(moveLateral) -> Compute CoM and Base Rotation References/4(moveLateral)
  Detect Robot Movement Request From Joystick/3(moveUpDown) -> Compute CoM and Base Rotation References/5(moveUpDown)
  Bus Selector/2 -> ForwardKinematics/2  "<jointPos>"
  "holder "/1 -> Selector1/1
  Detect Robot Movement Request From Joystick/1(moveFront) -> Compute CoM and Base Rotation References/3(moveFront)
  Detect Robot Movement Request From Joystick/7(turbo_mode) -> Compute CoM and Base Rotation References/9(turbo_mode)

== system momentumBasedFlying/FLYING CONTROLLER (CORE) V2.5/Flying State Machine/Compute Gains And References/Smooth CoM and Base References ==
  pos_vel_acc_jerk_CoM_des : Inport
  smoothingTimeCoMPos : Inport  Port=2
  gainSmoothingBaseRot : Inport  Port=3
  rot_vel_acc_jerk_base_des : Inport  Port=4
  Constant : Constant  Value=Config.references.SMOOTH_BASE_ROT_REFERENCES
  Constant1 : Constant  Value=Config.references.SMOOTH_COM_POS_REFERENCES
  Smooth Position References : Subsystem
  Smooth Reference Orientations : Subsystem
  Switch : Switch  Criteria=u2 > Threshold
  Switch2 : Switch  Criteria=u2 > Threshold
  pos_vel_acc_jerk_CoM_des_smooth : Outport  VectorParamsAs1DForOutWhenUnconnected=off
  rot_vel_acc_jerk_base_des_smooth : Outport  Port=2  VectorParamsAs1DForOutWhenUnconnected=off
  wires:
  Smooth Position References/1(pos_vel_acc_jerk_CoM_des_smooth) -> Switch/1
  smoothingTimeCoMPos/1 -> Smooth Position References/1(smoothingTimeCoMPos)
  pos_vel_acc_jerk_CoM_des/1 -> Switch/3, Smooth Position References/2(pos_vel_acc_jerk_CoM_des)
  Switch2/1 -> rot_vel_acc_jerk_base_des_smooth/1
  Switch/1 -> pos_vel_acc_jerk_CoM_des_smooth/1
  Constant1/1 -> Switch/2
  rot_vel_acc_jerk_base_des/1 -> Smooth Reference Orientations/1(rot_vel_acc_jerk_base_des)
  gainSmoothingBaseRot/1 -> Switch2/3, Smooth Reference Orientations/2(gainSmoothingBaseRot)
  Smooth Reference Orientations/1(rot_acc_vel_jerk_base_des_smooth) -> Switch2/1
  Constant/1 -> Switch2/2

== system momentumBasedFlying/FLYING CONTROLLER (CORE) V2.5/Dynamics and Kinematics/Dynamic Quantities/Momentum and CentroidalMomentum Matrix/CentroidalMomentum Matrix iCub 23//25 DoFs ==
  note: REQUIRED WORKSPACE PARAMETER:
      |
      | - Config.N_DOF: number of DoFs. Expected
      | values: either 23 or 25.
  w_H_b : Inport
  jointPos : Inport  Port=2
  CMM_base : Subsystem
  CMM_joints : Subsystem
  Combine CMM : Subsystem
  Constant : Constant  Value=eye(Config.N_DOF)
  Constant1 : Constant  Value=Config.N_DOF
  Constant2 : Constant  Value=Config.N_DOF
  Select CMM 23 or 25 : MATLAB Function  TreatAsAtomicUnit=on
  Selector Matrix : MATLAB Function  TreatAsAtomicUnit=on
  CMM : Outport  VectorParamsAs1DForOutWhenUnconnected=off
  wires:
  jointPos/1 -> CMM_base/2(jointPos), CMM_joints/2(jointPos)
  w_H_b/1 -> CMM_base/1(w_H_b), CMM_joints/1(w_H_b)
  Selector Matrix/1(SelMatrix) -> CMM_joints/3(SelMatrix)
  Constant1/1 -> Selector Matrix/1(ROBOT_DOF)
  Constant/1 -> Selector Matrix/2(SelMatrix_0)
  Combine CMM/1(CMM_25DoFs) -> Select CMM 23 or 25/1(CMM_25)
  CMM_base/1(CMM_base) -> Combine CMM/1(CMM_base)
  CMM_joints/1(CMM_joints_from_1_to_20) -> Combine CMM/2(CMM_joints_1_20)
  CMM_joints/2(CMM_group5_25DoFs) -> Combine CMM/3(CMM_group5_25DoFs)
  CMM_joints/3(CMM_group5_23DoFs) -> Combine CMM/4(CMM_group5_23DoFs)
  Constant2/1 -> Select CMM 23 or 25/2(N_DOF)
  Select CMM 23 or 25/1(CMM) -> CMM/1
  Combine CMM/2(CMM_23DoFs) -> Select CMM 23 or 25/3(CMM_23)

== system momentumBasedFlying/FLYING CONTROLLER (CORE) V2.5/Flight Controller RAL-HUMANOIDS V3.1- Aerodynamic Effects Compensation/Joint Torque Control for Flying/QP torqueControl/QP torqueControl - balancing ==
  H : Inport
  g : Inport  Port=2
  ub : Inport  Port=3
  lb : Inport  Port=4
  AEq : Inport  Port=5
  lbEq : Inport  Port=6
  ubEq : Inport  Port=7
  Enable : EnablePort
  Combine Bounds and Inequalities : MATLAB Function  TreatAsAtomicUnit=on
  MatchSignalSizes : WBToolboxLibrary/Utilities/MatchSignalSizes
      settings: SourceProductName=WholeBodyToolbox
  QP balancing-torqueControl : WBToolboxLibrary/Utilities/QP  lbA=on  ubA=on  lb=off  ub=off  computeObjVal=off  stopIfFails=off
      settings: SourceProductName=WholeBodyToolbox
  QPStatus_balancing : Outport  VectorParamsAs1DForOutWhenUnconnected=off
  QPOutput_balancing : Outport  Port=2  VectorParamsAs1DForOutWhenUnconnected=off
  wires:
  Combine Bounds and Inequalities/3(ubEq_combined) -> QP balancing-torqueControl/5
  Combine Bounds and Inequalities/2(lbEq_combined) -> QP balancing-torqueControl/4
  Combine Bounds and Inequalities/1(AEq_combined) -> QP balancing-torqueControl/3
  ub/1 -> Combine Bounds and Inequalities/5(ub)
  lb/1 -> Combine Bounds and Inequalities/4(lb)
  ubEq/1 -> Combine Bounds and Inequalities/3(ubEq)
  lbEq/1 -> Combine Bounds and Inequalities/2(lbEq)
  AEq/1 -> Combine Bounds and Inequalities/1(AEq)
  g/1 -> QP balancing-torqueControl/2, MatchSignalSizes/1
  H/1 -> QP balancing-torqueControl/1
  QP balancing-torqueControl/1 -> MatchSignalSizes/2
  MatchSignalSizes/1 -> QPOutput_balancing/1
  QP balancing-torqueControl/2 -> QPStatus_balancing/1

== system momentumBasedFlying/FLYING CONTROLLER (CORE) V2.5/Flight Controller RAL-HUMANOIDS V3.1- Aerodynamic Effects Compensation/Joint Torque Control for Flying/QP torqueControl/QP torqueControl - flight ==
  H : Inport
  g : Inport  Port=2
  ub : Inport  Port=3
  lb : Inport  Port=4
  Enable : EnablePort
  Constant : Constant  Value=eye(Config.N_DOF)
  MatchSignalSizes : WBToolboxLibrary/Utilities/MatchSignalSizes
      settings: SourceProductName=WholeBodyToolbox
  QP flight-torqueControl : WBToolboxLibrary/Utilities/QP  lbA=on  ubA=on  lb=off  ub=off  computeObjVal=off  stopIfFails=off
      settings: SourceProductName=WholeBodyToolbox
  QPStatus_flight : Outport  VectorParamsAs1DForOutWhenUnconnected=off
  QPOutput_flight : Outport  Port=2  VectorParamsAs1DForOutWhenUnconnected=off
  wires:
  ub/1 -> QP flight-torqueControl/5
  g/1 -> MatchSignalSizes/1, QP flight-torqueControl/2
  H/1 -> QP flight-torqueControl/1
  QP flight-torqueControl/1 -> MatchSignalSizes/2
  MatchSignalSizes/1 -> QPOutput_flight/1
  lb/1 -> QP flight-torqueControl/4
  QP flight-torqueControl/2 -> QPStatus_flight/1
  Constant/1 -> QP flight-torqueControl/3

== system momentumBasedFlying/FLYING CONTROLLER (CORE) V2.5/Flight Controller RAL-HUMANOIDS V3.1- Aerodynamic Effects Compensation/Joint Torque Control for Flying/QP torqueControl/Select QP torqueControl Output ==
  QPStatus_balancing : Inport
  QPOutput_balancing : Inport  Port=2
  feetContactIsActive : Inport  Port=3
  QPStatus_flight : Inport  Port=4
  QPOutput_flight : Inport  Port=5
  Demux : Demux  Outputs=[12;Config.N_DOF]
  Switch : Switch  Criteria=u2 > Threshold
  Switch1 : Switch  Criteria=u2 > Threshold
  contactForces_QP : Terminator
  jointTorques_star : Outport  VectorParamsAs1DForOutWhenUnconnected=off
  exitFlagQP_torqueControl : Outport  Port=2  VectorParamsAs1DForOutWhenUnconnected=off
  wires:
  Demux/2 -> Switch1/1
  Demux/1 -> contactForces_QP/1
  QPOutput_flight/1 -> Switch1/3
  QPOutput_balancing/1 -> Demux/1
  Switch/1 -> exitFlagQP_torqueControl/1
  QPStatus_flight/1 -> Switch/3
  QPStatus_balancing/1 -> Switch/1
  feetContactIsActive/1 -> Switch/2, Switch1/2
  Switch1/1 -> jointTorques_star/1

== system momentumBasedFlying/FLYING CONTROLLER (CORE) V2.5/Flight Controller RAL-HUMANOIDS V3.1- Aerodynamic Effects Compensation/Momentum Control for Flying/QP Solver and Integrate Contact Forces Derivative/Integrate the Contact Forces Derivative ==
  contactForcesDot_star : Inport
  contactForces : Inport  Port=2
  feetContactIsActive : Inport  Port=3
  Discrete-Time Integrator1 : DiscreteIntegrator  ExternalReset=either  InitialConditionSource=external  InitialCondition=zeros(6,1)  SampleTime=Config.tStep  ICPrevOutput=DiscIntNeverNeededParam  ICPrevScaledInput=DiscIntNeverNeededParam
  Select Integrator Initial Condition : MATLAB Function  TreatAsAtomicUnit=on
  deadZone : Subsystem
  contactForces_star : Outport  VectorParamsAs1DForOutWhenUnconnected=off
  tag scope: contactForcesDot_star=global
  wires:
  Select Integrator Initial Condition/1(contactForces_0) -> Discrete-Time Integrator1/3
  feetContactIsActive/1 -> Discrete-Time Integrator1/2, Select Integrator Initial Condition/1(feetContactIsActive)
  contactForces/1 -> Select Integrator Initial Condition/2(contactForces)
  deadZone/1(u_cut) -> Discrete-Time Integrator1/1
  contactForcesDot_star/1 -> [contactForcesDot_star], deadZone/1(u)
  Discrete-Time Integrator1/1 -> contactForces_star/1

== system momentumBasedFlying/FLYING CONTROLLER (CORE) V2.5/Flight Controller RAL-HUMANOIDS V3.1- Aerodynamic Effects Compensation/Momentum Control for Flying/QP Solver and Integrate Contact Forces Derivative/QP momentumControl ==
  HessianMatrixQP : Inport
  gVectorQP : Inport  Port=2
  lowerBoundQP : Inport  Port=3
  upperBoundQP : Inport  Port=4
  feetContactIsActive : Inport  Port=5
  NOT : Logic  Operator=NOT  IconShape=distinctive  AllPortsSameDT=off  OutDataTypeStr=boolean
  Process QP Inputs Momentum Control : MATLAB Function  TreatAsAtomicUnit=on
  QP momentumControl - balancing : Subsystem  TreatAsAtomicUnit=on
  QP momentumControl - flight : Subsystem  TreatAsAtomicUnit=on
  Select QP momentumControl Output : Subsystem
  jetsIntensitiesDot_star : Outport  VectorParamsAs1DForOutWhenUnconnected=off
  contactForcesDot_star : Outport  Port=2  VectorParamsAs1DForOutWhenUnconnected=off
  jointVel_star : Outport  Port=3  VectorParamsAs1DForOutWhenUnconnected=off
  exitFlagQP_momentumControl : Outport  Port=4  VectorParamsAs1DForOutWhenUnconnected=off
  wires:
  QP momentumControl - flight/2(QPOutput_flight) -> Select QP momentumControl Output/5(QPOutput_flight)
  QP momentumControl - flight/1(QPStatus_flight) -> Select QP momentumControl Output/4(QPStatus_flight)
  QP momentumControl - balancing/2(QPOutput_balancing) -> Select QP momentumControl Output/2(QPOutput_balancing)
  QP momentumControl - balancing/1(QPStatus_balancing) -> Select QP momentumControl Output/1(QPStatus_balancing)
  Select QP momentumControl Output/4(exitFlagQP_momentumControl) -> exitFlagQP_momentumControl/1
  NOT/1 -> QP momentumControl - flight/Enable
  Process QP Inputs Momentum Control/8(lb_flight) -> QP momentumControl - flight/4(lb)
  Process QP Inputs Momentum Control/7(ub_flight) -> QP momentumControl - flight/3(ub)
  Process QP Inputs Momentum Control/4(lb_balancing) -> QP momentumControl - balancing/4(lb)
  Process QP Inputs Momentum Control/3(ub_balancing) -> QP momentumControl - balancing/3(ub)
  Process QP Inputs Momentum Control/6(g_flight) -> QP momentumControl - flight/2(g)
  Process QP Inputs Momentum Control/5(H_flight) -> QP momentumControl - flight/1(H)
  Process QP Inputs Momentum Control/2(g_balancing) -> QP momentumControl - balancing/2(g)
  Process QP Inputs Momentum Control/1(H_balancing) -> QP momentumControl - balancing/1(H)
  Select QP momentumControl Output/2(contactForcesDot_star) -> contactForcesDot_star/1
  Select QP momentumControl Output/3(jointVel_star) -> jointVel_star/1
  Select QP momentumControl Output/1(jetsIntensitiesDot_star) -> jetsIntensitiesDot_star/1
  HessianMatrixQP/1 -> Process QP Inputs Momentum Control/1(HessianMatrixQP)
  upperBoundQP/1 -> Process QP Inputs Momentum Control/4(upperBoundQP)
  feetContactIsActive/1 -> QP momentumControl - balancing/Enable, NOT/1, Select QP momentumControl Output/3(feetContactIsActive)
  lowerBoundQP/1 -> Process QP Inputs Momentum Control/3(lowerBoundQP)
  gVectorQP/1 -> Process QP Inputs Momentum Control/2(gVectorQP)

== system momentumBasedFlying/FLYING CONTROLLER (CORE) V2.5/Flight Controller RAL-HUMANOIDS V3.1- Aerodynamic Effects Compensation/Momentum Control for Flying/extendedKalmanFilter4jets/EKF_jet1 ==
  input : Inport
  jetIntensityMeasurement : Inport  Port=2
  Constant : Constant  Value=[Config.initT, Config.initTdot]
  Constant1 : Constant  Value=Config.ekf.initP
  Discrete-Time Integrator1 : DiscreteIntegrator  InitialConditionSource=external  SampleTime=Config.tStep  ICPrevOutput=DiscIntNeverNeededParam  ICPrevScaledInput=DiscIntNeverNeededParam
  Discrete-Time Integrator2 : DiscreteIntegrator  InitialConditionSource=external  SampleTime=Config.tStep  ICPrevOutput=DiscIntNeverNeededParam  ICPrevScaledInput=DiscIntNeverNeededParam
  "EKF " : MATLAB Function  TreatAsAtomicUnit=on
  splitVector : MATLAB Function  TreatAsAtomicUnit=on
  jetIntensityFiltered : Outport  VectorParamsAs1DForOutWhenUnconnected=off
  jetDerivativeEstimated : Outport  Port=2  VectorParamsAs1DForOutWhenUnconnected=off
  wires:
  splitVector/2(x2) -> jetDerivativeEstimated/1
  splitVector/1(x1) -> jetIntensityFiltered/1
  Constant1/1 -> Discrete-Time Integrator2/2
  Discrete-Time Integrator2/1 -> "EKF "/4(P)
  jetIntensityMeasurement/1 -> "EKF "/3(measurement)
  Constant/1 -> Discrete-Time Integrator1/2
  Discrete-Time Integrator1/1 -> splitVector/1(x), "EKF "/1(x)
  input/1 -> "EKF "/2(input)
  "EKF "/1(xDot) -> Discrete-Time Integrator1/1
  "EKF "/2(Pdot) -> Discrete-Time Integrator2/1

== system momentumBasedFlying/FLYING CONTROLLER (CORE) V2.5/Flight Controller RAL-HUMANOIDS V3.1- Aerodynamic Effects Compensation/Momentum Control for Flying/extendedKalmanFilter4jets/EKF_jet2 ==
  input : Inport
  jetIntensityMeasurement : Inport  Port=2
  Constant : Constant  Value=[Config.initT, Config.initTdot]
  Constant1 : Constant  Value=Config.ekf.initP
  Discrete-Time Integrator1 : DiscreteIntegrator  InitialConditionSource=external  SampleTime=Config.tStep  ICPrevOutput=DiscIntNeverNeededParam  ICPrevScaledInput=DiscIntNeverNeededParam
  Discrete-Time Integrator2 : DiscreteIntegrator  InitialConditionSource=external  SampleTime=Config.tStep  ICPrevOutput=DiscIntNeverNeededParam  ICPrevScaledInput=DiscIntNeverNeededParam
  "EKF " : MATLAB Function  TreatAsAtomicUnit=on
  splitVector : MATLAB Function  TreatAsAtomicUnit=on
  jetIntensityFiltered : Outport  VectorParamsAs1DForOutWhenUnconnected=off
  jetDerivativeEstimated : Outport  Port=2  VectorParamsAs1DForOutWhenUnconnected=off
  wires:
  "EKF "/2(Pdot) -> Discrete-Time Integrator2/1
  "EKF "/1(xDot) -> Discrete-Time Integrator1/1
  input/1 -> "EKF "/2(input)
  Discrete-Time Integrator1/1 -> "EKF "/1(x), splitVector/1(x)
  Constant/1 -> Discrete-Time Integrator1/2
  jetIntensityMeasurement/1 -> "EKF "/3(measurement)
  Discrete-Time Integrator2/1 -> "EKF "/4(P)
  Constant1/1 -> Discrete-Time Integrator2/2
  splitVector/1(x1) -> jetIntensityFiltered/1
  splitVector/2(x2) -> jetDerivativeEstimated/1
